simulink library "cross_prod"  (R2020b)
settings: Solver=VariableStepAuto  StartTime=0.0  StopTime=10.0  RelTol=1e-3
settings Model: Creator=whitehole  LastModifiedBy=whitehole

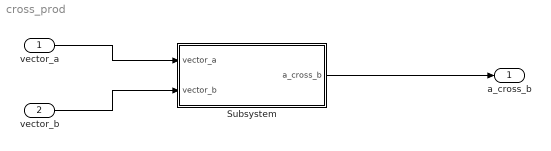
== system cross_prod ==
  vector_a : Inport
  vector_b : Inport  Port=2
  Subsystem : Subsystem
  a_cross_b : Outport
  wires:
  vector_a/1 -> Subsystem/1(vector_a)
  vector_b/1 -> Subsystem/2(vector_b)
  Subsystem/1(a_cross_b) -> a_cross_b/1

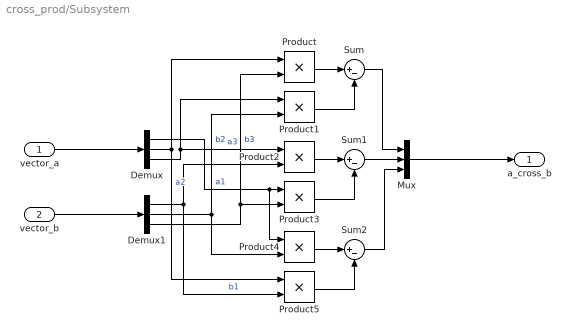
== system cross_prod/Subsystem ==
  vector_a : Inport
  vector_b : Inport  Port=2
  Demux : Demux  Outputs=3
  Demux1 : Demux  Outputs=3
  Mux : Mux  Inputs=3
  Product{,1..5} (6 alike) : Product
  Sum : Sum  Inputs=|+-
  Sum1 : Sum  Inputs=|+-
  Sum2 : Sum  Inputs=|+-
  a_cross_b : Outport
  wires:
  Demux1/2 -> Product4/2, Product1/2  "b2"
  Product/1 -> Sum/1
  Product2/1 -> Sum1/1
  Mux/1 -> a_cross_b/1
  vector_b/1 -> Demux1/1
  Demux1/1 -> Product5/2, Product2/2  "b1"
  Sum1/1 -> Mux/2
  Product5/1 -> Sum2/2
  Product3/1 -> Sum1/2
  Product4/1 -> Sum2/1
  Demux/1 -> Product4/1, Product3/1  "a1"
  Sum2/1 -> Mux/3
  Demux/2 -> Product5/1, Product/1  "a2"
  vector_a/1 -> Demux/1
  Demux/3 -> Product2/1, Product1/1  "a3"
  Sum/1 -> Mux/1
  Demux1/3 -> Product3/2, Product/2  "b3"
  Product1/1 -> Sum/2
